simulink library "avlAerodynamics6D_ul"  (R2022a)
settings: Solver=VariableStepAuto  StartTime=0.0  StopTime=10.0  RelTol=1e-3
undefined symbols (not defined in the file or in its folder): CLtotTbl
settings Model: Creator=mcobb  LastModifiedBy=lhill8
settings SolverCC: AlgebraicLoopSolver=TrustRegion
settings DebuggingCC: UnconnectedInputMsg=warning  UnconnectedOutputMsg=warning  UnconnectedLineMsg=warning  SFMachineParentedDataDiag=warning  ArithmeticOperatorsInVariantConditions=warning
settings SFSimCC: CustomCodeUndefinedFunction=UseInterfaceOnly

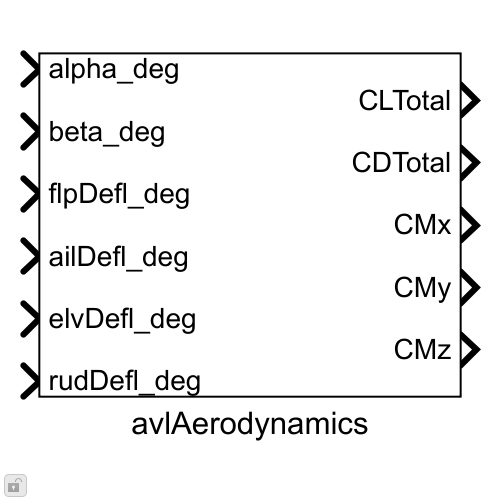
[thumbnail: Simulink's stored preview of the top-level diagram]
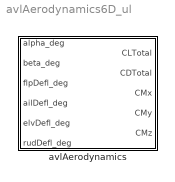
== system avlAerodynamics6D_ul ==
  avlAerodynamics : Subsystem  mask{CLTable=CLtotTbl, CDTable=CLtotTbl, CMxTable=CLtotTbl, CMyTable=CLtotTbl, CMzTable=CLtotTbl}
      mask prompts: CLTable "CL lookup table object"; CDTable "CD lookup table object"; CMxTable "CMx lookup table object"; CMyTable "CMy lookup table object"; CMzTable "CMz lookup table object"

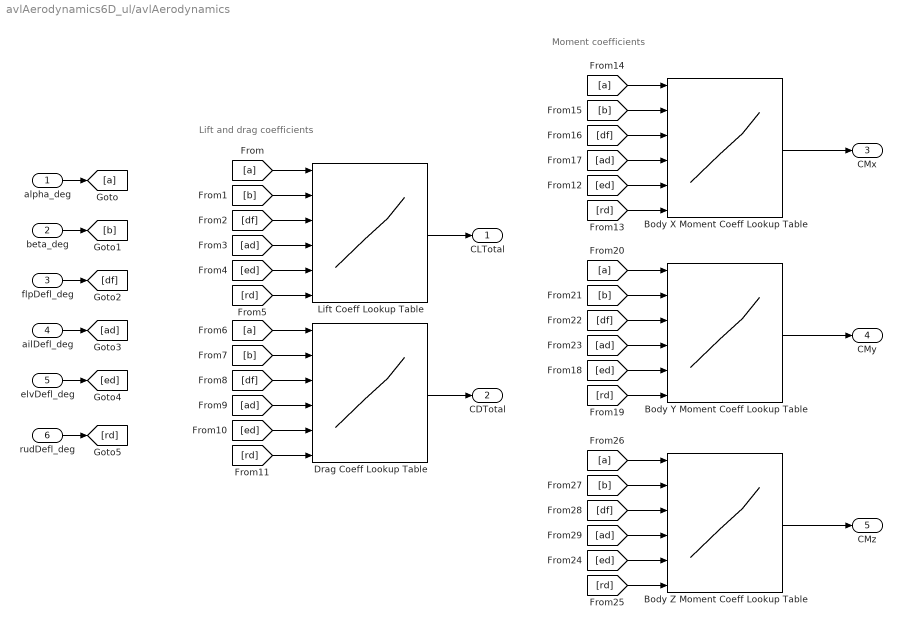
== system avlAerodynamics6D_ul/avlAerodynamics ==
  note: Moment coefficients
  note: Lift and drag coefficients
  alpha_deg : Inport
  beta_deg : Inport  Port=2
  flpDefl_deg : Inport  Port=3
  ailDefl_deg : Inport  Port=4
  elvDefl_deg : Inport  Port=5
  rudDefl_deg : Inport  Port=6
  Body X Moment Coeff Lookup Table : Lookup_n-D  NumberOfTableDimensions=6  DataSpecification=Lookup table object  LookupTableObject=CMxTable  BreakpointsForDimension3=[5, 7]  Table=reshape(repmat([4 5 6;16 19 20;10 18 23],1,2),[3,3,2])  InternalRulePriority=Speed  RndMeth=Simplest
      settings: InputPortMap=u0,u1,u2,u3,u4,u5
  Body Y Moment Coeff Lookup Table : Lookup_n-D  NumberOfTableDimensions=6  DataSpecification=Lookup table object  LookupTableObject=CMyTable  BreakpointsForDimension3=[5, 7]  Table=reshape(repmat([4 5 6;16 19 20;10 18 23],1,2),[3,3,2])  InternalRulePriority=Speed  RndMeth=Simplest
      settings: InputPortMap=u0,u1,u2,u3,u4,u5
  Body Z Moment Coeff Lookup Table : Lookup_n-D  NumberOfTableDimensions=6  DataSpecification=Lookup table object  LookupTableObject=CMzTable  BreakpointsForDimension3=[5, 7]  Table=reshape(repmat([4 5 6;16 19 20;10 18 23],1,2),[3,3,2])  InternalRulePriority=Speed  RndMeth=Simplest
      settings: InputPortMap=u0,u1,u2,u3,u4,u5
  Drag Coeff Lookup Table : Lookup_n-D  NumberOfTableDimensions=6  DataSpecification=Lookup table object  LookupTableObject=CDTable  BreakpointsForDimension3=[5, 7]  Table=reshape(repmat([4 5 6;16 19 20;10 18 23],1,2),[3,3,2])  InternalRulePriority=Speed  RndMeth=Simplest
      settings: InputPortMap=u0,u1,u2,u3,u4,u5
  Lift Coeff Lookup Table : Lookup_n-D  NumberOfTableDimensions=6  DataSpecification=Lookup table object  LookupTableObject=CLTable  BreakpointsForDimension3=[5, 7]  Table=reshape(repmat([4 5 6;16 19 20;10 18 23],1,2),[3,3,2])  InternalRulePriority=Speed  RndMeth=Simplest
      settings: InputPortMap=u0,u1,u2,u3,u4,u5
  CLTotal : Outport  VectorParamsAs1DForOutWhenUnconnected=off
  CDTotal : Outport  Port=2  VectorParamsAs1DForOutWhenUnconnected=off
  CMx : Outport  Port=3  VectorParamsAs1DForOutWhenUnconnected=off
  CMy : Outport  Port=4  VectorParamsAs1DForOutWhenUnconnected=off
  CMz : Outport  Port=5  VectorParamsAs1DForOutWhenUnconnected=off
  wires:
  alpha_deg/1 -> [a]
  beta_deg/1 -> [b]
  flpDefl_deg/1 -> [df]
  ailDefl_deg/1 -> [ad]
  elvDefl_deg/1 -> [ed]
  rudDefl_deg/1 -> [rd]
  [b] -> Lift Coeff Lookup Table/2
  [a] -> Lift Coeff Lookup Table/1
  [df] -> Lift Coeff Lookup Table/3
  [ad] -> Lift Coeff Lookup Table/4
  [ed] -> Lift Coeff Lookup Table/5
  [rd] -> Lift Coeff Lookup Table/6
  Lift Coeff Lookup Table/1 -> CLTotal/1
  [rd] -> Drag Coeff Lookup Table/6
  [ed] -> Drag Coeff Lookup Table/5
  [ad] -> Drag Coeff Lookup Table/4
  [df] -> Drag Coeff Lookup Table/3
  [a] -> Drag Coeff Lookup Table/1
  [b] -> Drag Coeff Lookup Table/2
  [b] -> Body X Moment Coeff Lookup Table/2
  [a] -> Body X Moment Coeff Lookup Table/1
  [df] -> Body X Moment Coeff Lookup Table/3
  [ad] -> Body X Moment Coeff Lookup Table/4
  [ed] -> Body X Moment Coeff Lookup Table/5
  [rd] -> Body X Moment Coeff Lookup Table/6
  [rd] -> Body Y Moment Coeff Lookup Table/6
  [ed] -> Body Y Moment Coeff Lookup Table/5
  [ad] -> Body Y Moment Coeff Lookup Table/4
  [df] -> Body Y Moment Coeff Lookup Table/3
  [a] -> Body Y Moment Coeff Lookup Table/1
  [b] -> Body Y Moment Coeff Lookup Table/2
  [b] -> Body Z Moment Coeff Lookup Table/2
  [a] -> Body Z Moment Coeff Lookup Table/1
  [df] -> Body Z Moment Coeff Lookup Table/3
  [ad] -> Body Z Moment Coeff Lookup Table/4
  [ed] -> Body Z Moment Coeff Lookup Table/5
  [rd] -> Body Z Moment Coeff Lookup Table/6
  Drag Coeff Lookup Table/1 -> CDTotal/1
  Body X Moment Coeff Lookup Table/1 -> CMx/1
  Body Y Moment Coeff Lookup Table/1 -> CMy/1
  Body Z Moment Coeff Lookup Table/1 -> CMz/1
